simulink model "SP_Dynamic_17Okt_ExergyFlow"  (R2019b)
settings: Solver=FixedStepAuto  StartTime=0.0  StopTime=0  FixedStep=1/3600  RelTol=1e-3
model workspace (MAT data in the model file):
  AD = Simulink.Parameter
  AD.Value = [1; 1; 1; 23.3; 33.9; 32.8; 49.9; 50.5]
  AD.DataType = 'auto'
  AD.Dimensions = [8 1]
  AG = Simulink.Parameter
  AG.Value = [3.411e-06; 3.799e-07; 2.491e-07; 3.567e-07; 3.463e-07; 3.93e-07; 1.7e-07; 1.5e-07]
  AG.Description = 'Coefficient A to determine Enthalpy
    | MBtu/lb·°F'
  AG.DataType = 'auto'
  AG.Dimensions = [8 1]
  AH = Simulink.Parameter
  AH.Value = [1e-06; 1e-06; 1e-06; 9.6e-07; 5.73e-07; 6.52e-07; 5.15e-07; 4.71e-07]
  AH.Description = 'Coefficient C to determine Enthalpy
    | MBtu/lb·°F³'
  AH.DataType = 'auto'
  AH.Dimensions = [8 1]
  AV = Simulink.Parameter
  AV.Value = [1e-06; 1e-06; 1e-06; 8.67e-05; 0.00016; 0.00016; 0.000225; 0.000209]
  AV.DataType = 'auto'
  AV.Dimensions = [8 1]
  AVP = Simulink.Parameter
  AVP.Value = [0; 0; 0; 15.92; 16.35; 16.35; 16.43; 17.21]
  AVP.DataType = 'auto'
  AVP.Dimensions = [8 1]
  BCHL = Simulink.Parameter
  BCHL.Value = [0; 0; 0; 2118895; 2331760; 2492349; 2279927; 2994129]
  BCHL.DataType = 'auto'
  BCHL.Dimensions = [8 1]
  BCHV = Simulink.Parameter
  BCHV.Value = [254278; 948838; 625079; 1822034; 1979455; 2321416; 1491254; 1822996]
  BCHV.DataType = 'auto'
  BCHV.Dimensions = [8 1]
  BD = Simulink.Parameter
  BD.Value = [0; 0; 0; -0.07; -0.0957; -0.0995; -0.0191; -0.0541]
  BD.DataType = 'auto'
  BD.Dimensions = [8 1]
  BG = Simulink.Parameter
  BG.Value = [7.18e-10; 1.08e-09; 1.36e-11; 8.51e-10; 8.96e-10; 1.02e-09; 0; 0]
  BG.Description = 'Coefficient B to determine Enthalpy
    | MBtu/lb·°F²'
  BG.DataType = 'auto'
  BG.Dimensions = [8 1]
  BH = Simulink.Parameter
  BH.Value = [0; 0; 0; 8.7e-09; 2.41e-09; 2.18e-09; 5.65e-10; 8.7e-10]
  BH.Description = 'Coefficient B to determine Enthalpy
    | MBtu/lb·°F²'
  BH.DataType = 'auto'
  BH.Dimensions = [8 1]
  BVP = Simulink.Parameter
  BVP.Value = [0; 0; 0; -1444; -2114; -2114; -2748; -3318]
  BVP.DataType = 'auto'
  BVP.Dimensions = [8 1]
  CD = Simulink.Parameter
  CD.Value = [0; 0; 0; -0.0002; -0.000152; -0.000233; -0.000425; -0.00015]
  CD.DataType = 'auto'
  CD.Dimensions = [8 1]
  CG = Simulink.Parameter
  CG.Value = [6e-13; -3.98e-13; -3.93e-14; -3.12e-13; -3.27e-13; -3.12e-13; 0; 0]
  CG.DataType = 'auto'
  CG.Dimensions = [8 1]
  CH = Simulink.Parameter
  CH.Value = [0; 0; 0; 4.81e-11; 1.82e-11; 1.94e-11; 3.82e-12; 2.62e-12]
  CH.DataType = 'auto'
  CH.Dimensions = [8 1]
  CVP = Simulink.Parameter
  CVP.Value = [0; 0; 0; 259; 265.5; 265.5; 232.9; 249.6]
  CVP.DataType = 'auto'
  CVP.Dimensions = [8 1]
  XMW = Simulink.Parameter
  XMW.Value = [2; 25.4; 28; 32; 46; 48; 62; 76]
  XMW.Description = 'Molecular Weight of components lb/lb-mol'
  XMW.DataType = 'auto'
  XMW.Dimensions = [8 1]
undefined symbols (not defined in the file or in its folder): magnitude, SETPT, XMEAS, XMV
libraries: mylib x165, dspindex x17
(part 1 of 10)
settings Model: Creator=j3vos  LastModifiedBy=j3vos
settings DataIOCC: ReturnWorkspaceOutputs=off
settings DebuggingCC: ArithmeticOperatorsInVariantConditions=warning
settings SFSimCC: SimUseLocalCustomCode=off  CustomCodeUndefinedFunction=UseInterfaceOnly
settings RTWCC: RTWUseLocalCustomCode=off

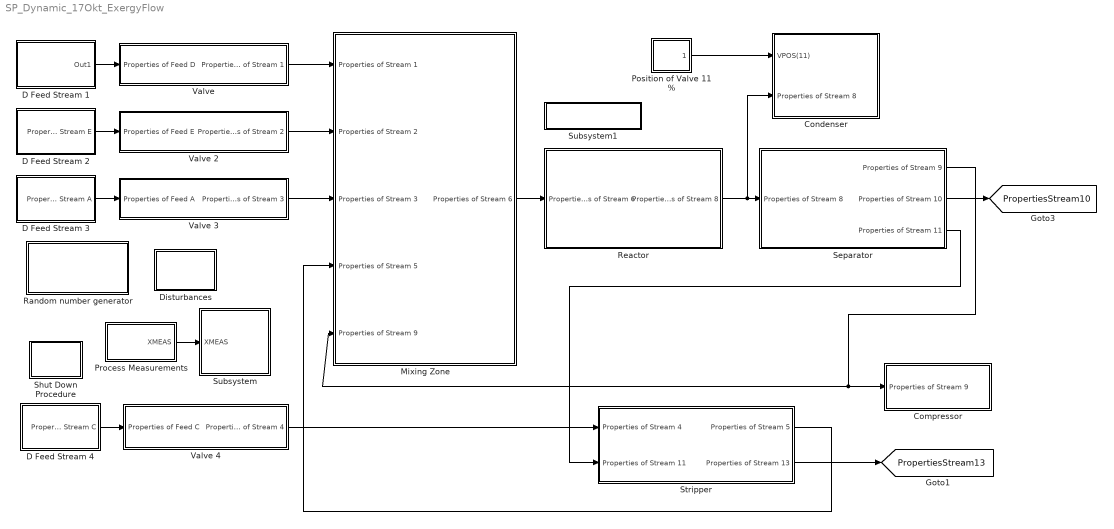
== system SP_Dynamic_17Okt_ExergyFlow ==
  Compressor : Subsystem
  Condenser : Subsystem
  D Feed Stream 1 : Subsystem  mask{XST1_A=0, XST1_B=0.0001, XST1_C=0, XST1_D=0.9999, XST1_E=0, XST1_F=0, XST1_G=0, XST1_H=0, TST1=45, VRNG1=400}
      mask prompts: XST1_A "Fraction of A in Stream 1"; XST1_B "Fraction of B in Stream 1"; XST1_C "Fraction of C in Stream 1"; XST1_D "Fraction of D in Stream 1"; XST1_E "Fraction of E in Stream 1"; XST1_F "Fraction of F in Stream 1"; XST1_G "Fraction of G in Stream 1"; XST1_H "Fraction of H in Stream 1"; TST1 "Temperature of Stream 1"; VRNG1 "Maximum flow of Stream 1"
      mask DialogControl DescTextVar Prompt: Enter the Composition, Temperature and Mass Flow of Feed Stream D entering the plant
      mask DialogControl ParameterGroupVar Prompt: Properties of Feed Stream D
      mask Display: color('Blue'),disp('Properties\nof\nFeed Stream D'),
  D Feed Stream 2 : Subsystem  mask{XST2_A=0, XST2_B=0, XST2_C=0, XST2_D=0, XST2_E=0.9999, XST2_F=0.0001, XST2_G=0, XST2_H=0, TST2=45, VRNG2=400}
      mask prompts: XST2_A "Fraction of A in Stream 2"; XST2_B "Fraction of B in Stream 2"; XST2_C "Fraction of C in Stream 2"; XST2_D "Fraction of D in Stream 2"; XST2_E "Fraction of E in Stream 2"; XST2_F "Fraction of F in Stream 2"; XST2_G "Fraction of G in Stream 2"; XST2_H "Fraction of H in Stream 2"; TST2 "Temperature of Stream 2"; VRNG2 "Maximum flow of Stream 2"
      mask DialogControl DescTextVar Prompt: Enter the Composition, Temperature and Mass Flow of Feed Stream E entering the plant
      mask DialogControl ParameterGroupVar Prompt: Properties of Feed Stream E
      mask Display: color('Red'),disp('Properties\nof\nFeed Stream E')
  D Feed Stream 3 : Subsystem  mask{XST3_A=0.9999, XST3_B=0.0001, XST3_C=0, XST3_D=0, XST3_E=0, XST3_F=0, XST3_G=0, XST3_H=0, TST3=45, VRNG3=100}
      mask prompts: XST3_A "Fraction of A in Stream 3"; XST3_B "Fraction of B in Stream 3"; XST3_C "Fraction of C in Stream 3"; XST3_D "Fraction of D in Stream 3"; XST3_E "Fraction of E in Stream 3"; XST3_F "Fraction of F in Stream 3"; XST3_G "Fraction of G in Stream 3"; XST3_H "Fraction of H in Stream 3"; TST3 "Temperature of Stream 3"; VRNG3 "Maximum flow of Stream 3"
      mask DialogControl DescTextVar Prompt: Enter the Composition, Temperature and Mass Flow of Feed Stream A entering the plant
      mask DialogControl ParameterGroupVar Prompt: Properties of Feed Stream A
      mask Display: color('Green'),disp('Properties\nof\nFeed Stream A')
  D Feed Stream 4 : Subsystem  mask{XST4_A=0.485, XST4_B=0.005, XST4_C=0.51, XST4_D=0, XST4_E=0, XST4_F=0, XST4_G=0, XST4_H=0, TST4=45, VRNG4=1500}
      mask prompts: XST4_A "Fraction of A in Stream 4"; XST4_B "Fraction of B in Stream 4"; XST4_C "Fraction of C in Stream 4"; XST4_D "Fraction of D in Stream 4"; XST4_E "Fraction of E in Stream 4"; XST4_F "Fraction of F in Stream 4"; XST4_G "Fraction of G in Stream 4"; XST4_H "Fraction of H in Stream 4"; TST4 "Temperature of Stream 4"; VRNG4 "Maximum flow of Stream 4"
      mask DialogControl DescTextVar Prompt: Enter the Composition, Temperature and Mass Flow of Feed Stream C entering the plant
      mask DialogControl ParameterGroupVar Prompt: Properties of Feed Stream C
      mask Display: color('Orange'),disp('Properties\nof\nFeed Stream C')
  Disturbances : Subsystem  mask{dd=1, IDV1=off, IDV2=off, IDV3=off, IDV4=off, IDV5=off, IDV6=off, IDV7=off, IDV8=off, IDV9=off, IDV10=off, IDV11=off, IDV12=off, IDV13=off, IDV14=off, IDV15=off, IDV16=off, IDV17=off, IDV18=off, IDV19=off, IDV20=off}
      mask prompts: dd "Simulation time when disturbances should be introduced"; IDV1 "IDV(1) - A/C feed ratio"; IDV2 "IDV(2) - B composition"; IDV3 "IDV(3) - D feed temperature"; IDV4 "IDV(4) - Reactor cooling water inlet temperature"; IDV5 "IDV(5) - Condenser cooling water inlet temperature"; IDV6 "IDV(6) - A feed loss"; IDV7 "IDV(7) - C header pressure loss (reduced availability)"; IDV8 "IDV(8) - A, B, C feed composition"; IDV9 "IDV(9) - D feed temperature"; IDV10 "IDV(10) - C feed temperature"; IDV11 "IDV(11) - Reactor cooling water inlet temperature"; IDV12 "IDV(12) - Condenser cooling water inlet temperature"; IDV13 "IDV(13) - Reaction kinetics"; IDV14 "IDV(14) - Reactor cooling water valve"; IDV15 "IDV(15) - Condenser cooling water valve"; IDV16 "IDV(16) - Unknown"; IDV17 "IDV(17) - Unknown"; IDV18 "IDV(18) - Unknown"; IDV19 "IDV(19) - Unknown"; IDV20 "IDV(20) - Unknown"
      mask DialogControl DescTextVar Prompt: Indicate if any disturbances are present (more than one can be ticked at a time)
      mask DialogControl ParameterGroupVar Prompt: Disturbances
      mask Display: color('Black'),disp('Disturbance\noff/on')
  Mixing Zone : Subsystem
  Position of Valve 11 % : Subsystem
  Process Measurements : Subsystem
  Random number generator : Subsystem  mask{gain_val=8322308324}
      mask prompts: gain_val "Random Number"
      mask init:
      | Gain=gain_val
      mask DialogControl DescTextVar Prompt: Enter a random number so that every runs results will differ
      mask DialogControl ParameterGroupVar Prompt: Random number generator
      mask Display: disp(['Random number:\n \n ',num2str(Gain)])
  Reactor : Subsystem
  Separator : Subsystem
  Shut Down Procedure : Subsystem
  Stripper : Subsystem
  Subsystem : Subsystem  mask{OPL=off, B=on, R=off, XMV1_0=63.05263039, XMV2_0=53.97970677, XMV3_0=24.64355755, XMV4_0=61.30192144, XMV5_0=22.21000000, XMV6_0=40.06374673, XMV7_0=38.10034370, XMV8_0=46.53415582, XMV9_0=47.44573456, XMV10_0=41.10581288, XMV11_0=18.11349055, XMV12_0=50.00000000}
      mask prompts: OPL "Open loop"; B "Braatz"; R "Ricker"; XMV1_0 "Initial value of XMV(1) - D Feed flow valve"; XMV2_0 "Initial value of XMV(2) - E Feed flow valve"; XMV3_0 "Initial value of XMV(3) - A Feed flow valve"; XMV4_0 "Initial value of XMV(4) - A and C Feed flow valve"; XMV5_0 "Initial value of XMV(5) - Compressor recycle valve"; XMV6_0 "Initial value of XMV(6) - Purge valve"; XMV7_0 "Initial value of XMV(7) - Separator liquid flow valve"; XMV8_0 "Initial value of XMV(8) - Stripper liquid product flow valve"; XMV9_0 "Initial value of XMV(9) - Stripper steam valve"; XMV10_0 "Initial value of XMV(10) - Reactor cooling water flow valve"; XMV11_0 "Initial value of XMV(11) - Condenser cooling water flow valve"; XMV12_0 "Initial value of XMV(12) - Agitator speed"
      mask DialogControl DescGroupVar Prompt: Manipulated variables
      mask DialogControl DescTextVar Prompt: Control loops for manipulated variables. Open loop is the original TEP process without any control. Only one loop can be selected for a run. The base case values are the initial values of the manipulated variables
      mask DialogControl ParameterGroupVar Prompt: Control strategy
      mask DialogControl Container6 Prompt: Base case values
      mask Display: color('Black'),disp('Control loop')
  Subsystem1 : Subsystem
      mask Display: color('Black'),disp('Exergy of streams')
  Valve : Subsystem
  Valve 2 : Subsystem
  Valve 3 : Subsystem
  Valve 4 : Subsystem
  tag scope: PropertiesStream10=global, PropertiesStream13=global
  wires:
  Position of Valve 11 %/1("YY(49) ") -> Condenser/1(VPOS(11))
  Valve/1(Properties of Stream 1) -> Mixing Zone/1(Properties of Stream 1)
  D Feed Stream 2/1("Properties of Feed Stream E ") -> Valve 2/1(Properties of Feed E)
  Valve 2/1(Properties of Stream 2) -> Mixing Zone/2(Properties of Stream 2)
  D Feed Stream 3/1("Properties of Feed Stream A ") -> Valve 3/1(Properties of Feed A)
  Valve 3/1(Properties of Stream 3) -> Mixing Zone/3(Properties of Stream 3)
  Stripper/1(Properties of Stream 5) -> Mixing Zone/4(Properties of Stream 5)
  Mixing Zone/1(Properties of Stream 6) -> Reactor/1(Properties of Stream 6)
  D Feed Stream 4/1("Properties of Feed Stream C ") -> Valve 4/1(Properties of Feed C)
  Valve 4/1(Properties of Stream 4) -> Stripper/1(Properties of Stream 4)
  Separator/3(Properties of Stream 11) -> Stripper/2(Properties of Stream 11)
  Reactor/1(Properties of Stream 8) -> Condenser/2(Properties of Stream 8), Separator/1(Properties of Stream 8)
  Separator/1(Properties of Stream 9) -> Mixing Zone/5(Properties of Stream 9), Compressor/1(Properties of Stream 9)
  D Feed Stream 1/1(Out1) -> Valve/1(Properties of Feed D)
  Process Measurements/1(XMEAS) -> Subsystem/1(XMEAS)
  Stripper/2(Properties of Stream 13) -> [PropertiesStream13]
  Separator/2(Properties of Stream 10) -> [PropertiesStream10]

== system SP_Dynamic_17Okt_ExergyFlow/Compressor ==
  Properties of Stream 9 : Inport
  "  " : Subsystem
  Bus Selector : BusSelector  OutputSignals=XMWS(9)
  CPDH Compressor work MBtu/h : Subsystem
  CPFLMX : Constant  Value=280275
  Subsystem : Subsystem
  Subsystem1 : Subsystem
  TKS Temperature of Separator K : Sum
  To Convert °C to K : Constant  Value=273.15
  tag scope: CPDH=global, FLMS=global
  wires:
  Subsystem1/1(FLCOEF) -> "  "/3(FLCOEF)
  Subsystem/1(PR) -> "  "/1(PR)
  CPFLMX/1 -> "  "/2(CPFLMX), Subsystem1/1(CPFLMX)
  CPDH Compressor work MBtu/h/1(CPDH) -> [CPDH]
  "  "/1(FLMS) -> [FLMS], CPDH Compressor work MBtu/h/1(FLMS)
  TKS Temperature of Separator K/1 -> CPDH Compressor work MBtu/h/2(TKS)
  [TCS] -> TKS Temperature of Separator K/1
  To Convert °C to K/1 -> TKS Temperature of Separator K/2
  Properties of Stream 9/1 -> Bus Selector/1
  Bus Selector/1 -> CPDH Compressor work MBtu/h/3("XMWS(9) ")  "<XMWS(9)>"

== system SP_Dynamic_17Okt_ExergyFlow/Condenser ==
  VPOS(11) : Inport
  Properties of Stream 8 : Inport  Port=2
  FWS Flow of cooling water to Condenser lb-mol/h : Subsystem
  Subsystem : Subsystem
  Subsystem1 : Subsystem
  "VRNG(11) Max flow of water through valve " : Constant  Value=1200
  tag scope: QUS=global
  wires:
  "VRNG(11) Max flow of water through valve "/1 -> FWS Flow of cooling water to Condenser lb-mol/h/2(VRNG(11))
  FWS Flow of cooling water to Condenser lb-mol/h/1(FWS) -> Subsystem1/1(FWS)
  VPOS(11)/1 -> FWS Flow of cooling water to Condenser lb-mol/h/1(VPOS(11))
  Subsystem/1("QUS ") -> Subsystem1/2(QUS), [QUS]
  Properties of Stream 8/1 -> Subsystem/1(Properties of Stream 8)
  Subsystem1/1("YY(38) ") -> Subsystem/2(In2)

== system SP_Dynamic_17Okt_ExergyFlow/D Feed Stream 1 ==
  Bus Creator : BusCreator  Inputs=4
  HST(1) Molar Enthalpy of Stream 1 MBtu/lb-mol : Subsystem
  TST(1) Temperature of Stream 1 °C : Subsystem
  VRNG(1) Max flow of Stream 1 through valve lb-mol/h : Constant  Value=VRNG1
  XST(I,1) Composition of Stream 1 : Constant  Value=[XST1_A;XST1_B;XST1_C;XST1_D;XST1_E;XST1_F;XST1_G;XST1_H]
  Out1 : Outport  VectorParamsAs1DForOutWhenUnconnected=off
  wires:
  XST(I,1) Composition of Stream 1/1 -> HST(1) Molar Enthalpy of Stream 1 MBtu/lb-mol/2(XST(I,1)), Bus Creator/1  "XST(I;1)"
  VRNG(1) Max flow of Stream 1 through valve lb-mol/h/1 -> Bus Creator/3  "VRNG(1)"
  HST(1) Molar Enthalpy of Stream 1 MBtu/lb-mol/1(HST(1)) -> Bus Creator/4  "HST(1)"
  TST(1) Temperature of Stream 1 °C/1(TST(1)) -> Bus Creator/2, HST(1) Molar Enthalpy of Stream 1 MBtu/lb-mol/1(TST(1))
  Bus Creator/1 -> Out1/1

== system SP_Dynamic_17Okt_ExergyFlow/D Feed Stream 2 ==
  Bus Creator : BusCreator  Inputs=4
  HST(2) Molar Enthalpy of Stream 2 MBtu/lb-mol : Subsystem
  TST(2) Temperature of Stream 2 °C : Constant  Value=TST2
  VRNG(2) Max flow of Stream 2 through valve lb-mol/h : Constant  Value=VRNG2
  XST(I,2) Composition of Stream 2 : Constant  Value=[XST2_A;XST2_B;XST2_C;XST2_D;XST2_E;XST2_F;XST2_G;XST2_H]
  "Properties of Feed Stream E " : Outport  VectorParamsAs1DForOutWhenUnconnected=off
  wires:
  XST(I,2) Composition of Stream 2/1 -> HST(2) Molar Enthalpy of Stream 2 MBtu/lb-mol/2(XST(I,2)), Bus Creator/1  "XST(I;2)"
  TST(2) Temperature of Stream 2 °C/1 -> HST(2) Molar Enthalpy of Stream 2 MBtu/lb-mol/1(TST(2)), Bus Creator/2  "TST(2)"
  VRNG(2) Max flow of Stream 2 through valve lb-mol/h/1 -> Bus Creator/3  "VRNG(2)"
  Bus Creator/1 -> "Properties of Feed Stream E "/1
  HST(2) Molar Enthalpy of Stream 2 MBtu/lb-mol/1(HST(2)) -> Bus Creator/4  "HST(2)"

== system SP_Dynamic_17Okt_ExergyFlow/D Feed Stream 3 ==
  Bus Creator : BusCreator  Inputs=4
  HST(3) Molar Enthalpy of Stream 3 MBtu/lb-mol : Subsystem
  TST(3) Temperature of Stream 3 °C : Constant  Value=TST3
  VRNG(3) Max flow of Stream 3 through valve lb-mol/h : Constant  Value=VRNG3
  XST(I,3) Composition of Stream 3 : Constant  Value=[XST3_A;XST3_B;XST3_C;XST3_D;XST3_E;XST3_F;XST3_G;XST3_H]
  "Properties of Feed Stream A " : Outport  VectorParamsAs1DForOutWhenUnconnected=off
  wires:
  XST(I,3) Composition of Stream 3/1 -> HST(3) Molar Enthalpy of Stream 3 MBtu/lb-mol/2(XST(I,3)), Bus Creator/1  "XST(I;3)"
  TST(3) Temperature of Stream 3 °C/1 -> HST(3) Molar Enthalpy of Stream 3 MBtu/lb-mol/1(TST(3)), Bus Creator/2  "TST(3)"
  VRNG(3) Max flow of Stream 3 through valve lb-mol/h/1 -> Bus Creator/3  "VRNG(3)"
  HST(3) Molar Enthalpy of Stream 3 MBtu/lb-mol/1(HST(3)) -> Bus Creator/4  "HST(3)"
  Bus Creator/1 -> "Properties of Feed Stream A "/1

== system SP_Dynamic_17Okt_ExergyFlow/D Feed Stream 4 ==
  note: TST(4)
      | Temperature of Stream 4
      | °C
  Bus Creator : BusCreator  Inputs=4
  Bus Selector : BusSelector  OutputSignals=TESUB8(1),TESUB8(2)
  Bus Selector1 : BusSelector  OutputSignals=IDV(1),IDV(2)
  Bus Selector2 : BusSelector  OutputSignals=TESUB8(4)
  Gain : Gain
  HST(4) Molar Enthalpy of Stream 4 MBtu/lb-mol : Subsystem
  VRNG(4) Max flow of Stream 4 through valve lb-mol/h : Constant  Value=VRNG4
  "XST(I;4) Composition of Stream 4 " : Subsystem
  "Properties of Feed Stream C " : Outport  VectorParamsAs1DForOutWhenUnconnected=off
  wires:
  "XST(I;4) Composition of Stream 4 "/1(XST(I;4)) -> HST(4) Molar Enthalpy of Stream 4 MBtu/lb-mol/2(XST(I,4)), Bus Creator/1  "XST(I;4)"
  Bus Selector2/1 -> HST(4) Molar Enthalpy of Stream 4 MBtu/lb-mol/1(TST(4)), Gain/1  "<TESUB8(4)>"
  VRNG(4) Max flow of Stream 4 through valve lb-mol/h/1 -> Bus Creator/3  "VRNG(4)"
  Bus Creator/1 -> "Properties of Feed Stream C "/1
  HST(4) Molar Enthalpy of Stream 4 MBtu/lb-mol/1(HST(4)) -> Bus Creator/4  "HST(4)"
  Bus Selector/2 -> "XST(I;4) Composition of Stream 4 "/2(TESUB8(2))  "<TESUB8(2)>"
  [TESUB8] -> Bus Selector2/1, Bus Selector/1
  Bus Selector/1 -> "XST(I;4) Composition of Stream 4 "/1(TESUB8(1))  "<TESUB8(1)>"
  [IDV] -> Bus Selector1/1
  Bus Selector1/1 -> "XST(I;4) Composition of Stream 4 "/3(IDV(1))  "<IDV(1)>"
  Bus Selector1/2 -> "XST(I;4) Composition of Stream 4 "/4(IDV(2))  "<IDV(2)>"
  Gain/1 -> Bus Creator/2  "TST(4)"

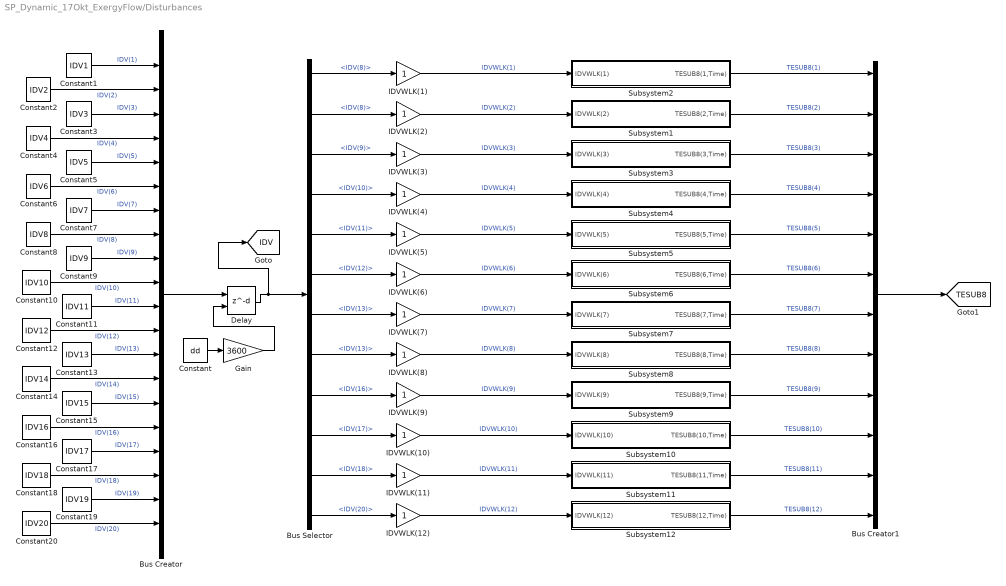
== system SP_Dynamic_17Okt_ExergyFlow/Disturbances ==
  Bus Creator : BusCreator  Inputs=20
  Bus Creator1 : BusCreator  Inputs=12
  Bus Selector : BusSelector  OutputSignals=IDV(8),IDV(8),IDV(9),IDV(10),IDV(11),IDV(12),IDV(13),IDV(13),IDV(16),IDV(17),IDV(18),IDV(20)
  Constant : Constant  Value=dd
  Constant1 : Constant  Value=IDV1
  Constant10 : Constant  Value=IDV10
  Constant11 : Constant  Value=IDV11
  Constant12 : Constant  Value=IDV12
  Constant13 : Constant  Value=IDV13
  Constant14 : Constant  Value=IDV14
  Constant15 : Constant  Value=IDV15
  Constant16 : Constant  Value=IDV16
  Constant17 : Constant  Value=IDV17
  Constant18 : Constant  Value=IDV18
  Constant19 : Constant  Value=IDV19
  Constant2 : Constant  Value=IDV2
  Constant20 : Constant  Value=IDV20
  Constant3 : Constant  Value=IDV3
  Constant4 : Constant  Value=IDV4
  Constant5 : Constant  Value=IDV5
  Constant6 : Constant  Value=IDV6
  Constant7 : Constant  Value=IDV7
  Constant8 : Constant  Value=IDV8
  Constant9 : Constant  Value=IDV9
  Delay : Delay  DelayLengthSource=Input port  DelayLength=1  DelayLengthUpperLimit=dd*3600  InitialCondition=0
      settings: InputPortMap=u0,p1
  Gain : Gain  Gain=3600
  IDVWLK(1) : Gain
  IDVWLK(10) : Gain
  IDVWLK(11) : Gain
  IDVWLK(12) : Gain
  IDVWLK(2) : Gain
  IDVWLK(3) : Gain
  IDVWLK(4) : Gain
  IDVWLK(5) : Gain
  IDVWLK(6) : Gain
  IDVWLK(7) : Gain
  IDVWLK(8) : Gain
  IDVWLK(9) : Gain
  Subsystem1 : Subsystem
  Subsystem10 : Subsystem
  Subsystem11 : Subsystem
  Subsystem12 : Subsystem
  Subsystem2 : Subsystem
  Subsystem3 : Subsystem
  Subsystem4 : Subsystem
  Subsystem5 : Subsystem
  Subsystem6 : Subsystem
  Subsystem7 : Subsystem
  Subsystem8 : Subsystem
  Subsystem9 : Subsystem
  tag scope: IDV=global, TESUB8=global
  wires:
  Constant1/1 -> Bus Creator/1  "IDV(1)"
  Constant2/1 -> Bus Creator/2  "IDV(2)"
  Constant3/1 -> Bus Creator/3  "IDV(3)"
  Constant4/1 -> Bus Creator/4  "IDV(4)"
  Constant5/1 -> Bus Creator/5  "IDV(5)"
  Constant6/1 -> Bus Creator/6  "IDV(6)"
  Constant7/1 -> Bus Creator/7  "IDV(7)"
  Constant8/1 -> Bus Creator/8  "IDV(8)"
  Constant9/1 -> Bus Creator/9  "IDV(9)"
  Constant10/1 -> Bus Creator/10  "IDV(10)"
  Constant11/1 -> Bus Creator/11  "IDV(11)"
  Constant12/1 -> Bus Creator/12  "IDV(12)"
  Constant13/1 -> Bus Creator/13  "IDV(13)"
  Constant14/1 -> Bus Creator/14  "IDV(14)"
  Constant15/1 -> Bus Creator/15  "IDV(15)"
  Constant16/1 -> Bus Creator/16  "IDV(16)"
  Constant17/1 -> Bus Creator/17  "IDV(17)"
  Constant18/1 -> Bus Creator/18  "IDV(18)"
  Constant19/1 -> Bus Creator/19  "IDV(19)"
  Constant20/1 -> Bus Creator/20  "IDV(20)"
  Bus Selector/5 -> IDVWLK(5)/1  "<IDV(11)>"
  Bus Selector/7 -> IDVWLK(7)/1  "<IDV(13)>"
  Bus Selector/9 -> IDVWLK(9)/1  "<IDV(16)>"
  Subsystem6/1(TESUB8(6,Time)) -> Bus Creator1/6  "TESUB8(6)"
  Subsystem3/1(TESUB8(3,Time)) -> Bus Creator1/3  "TESUB8(3)"
  Subsystem2/1(TESUB8(1,Time)) -> Bus Creator1/1  "TESUB8(1)"
  IDVWLK(10)/1 -> Subsystem10/1(IDVWLK(10))  "IDVWLK(10)"
  Subsystem7/1(TESUB8(7,Time)) -> Bus Creator1/7  "TESUB8(7)"
  Bus Selector/2 -> IDVWLK(2)/1  "<IDV(8)>"
  Subsystem8/1(TESUB8(8,Time)) -> Bus Creator1/8  "TESUB8(8)"
  Subsystem4/1(TESUB8(4,Time)) -> Bus Creator1/4  "TESUB8(4)"
  Bus Creator1/1 -> [TESUB8]
  Subsystem1/1(TESUB8(2,Time)) -> Bus Creator1/2  "TESUB8(2)"
  Bus Selector/12 -> IDVWLK(12)/1  "<IDV(20)>"
  IDVWLK(6)/1 -> Subsystem6/1(IDVWLK(6))  "IDVWLK(6)"
  IDVWLK(3)/1 -> Subsystem3/1(IDVWLK(3))  "IDVWLK(3)"
  IDVWLK(1)/1 -> Subsystem2/1(IDVWLK(1))  "IDVWLK(1)"
  Subsystem5/1(TESUB8(5,Time)) -> Bus Creator1/5  "TESUB8(5)"
  IDVWLK(9)/1 -> Subsystem9/1(IDVWLK(9))  "IDVWLK(9)"
  Bus Selector/1 -> IDVWLK(1)/1  "<IDV(8)>"
  Bus Selector/6 -> IDVWLK(6)/1  "<IDV(12)>"
  Bus Selector/4 -> IDVWLK(4)/1  "<IDV(10)>"
  IDVWLK(5)/1 -> Subsystem5/1(IDVWLK(5))  "IDVWLK(5)"
  Bus Selector/8 -> IDVWLK(8)/1  "<IDV(13)>"
  IDVWLK(2)/1 -> Subsystem1/1(IDVWLK(2))  "IDVWLK(2)"
  IDVWLK(8)/1 -> Subsystem8/1(IDVWLK(8))  "IDVWLK(8)"
  Bus Selector/3 -> IDVWLK(3)/1  "<IDV(9)>"
  Bus Selector/10 -> IDVWLK(10)/1  "<IDV(17)>"
  IDVWLK(7)/1 -> Subsystem7/1(IDVWLK(7))  "IDVWLK(7)"
  Bus Selector/11 -> IDVWLK(11)/1  "<IDV(18)>"
  Subsystem9/1(TESUB8(9,Time)) -> Bus Creator1/9  "TESUB8(9)"
  IDVWLK(4)/1 -> Subsystem4/1(IDVWLK(4))  "IDVWLK(4)"
  Bus Creator/1 -> Delay/1
  Subsystem10/1(TESUB8(10,Time)) -> Bus Creator1/10  "TESUB8(10)"
  Subsystem11/1(TESUB8(11,Time)) -> Bus Creator1/11  "TESUB8(11)"
  IDVWLK(11)/1 -> Subsystem11/1(IDVWLK(11))  "IDVWLK(11)"
  Subsystem12/1(TESUB8(12,Time)) -> Bus Creator1/12  "TESUB8(12)"
  IDVWLK(12)/1 -> Subsystem12/1(IDVWLK(12))  "IDVWLK(12)"
  Delay/1 -> Bus Selector/1, [IDV]
  Constant/1 -> Gain/1
  Gain/1 -> Delay/2

== system SP_Dynamic_17Okt_ExergyFlow/Mixing Zone ==
  Properties of Stream 1 : Inport
  Properties of Stream 2 : Inport  Port=2
  Properties of Stream 3 : Inport  Port=3
  Properties of Stream 5 : Inport  Port=4
  Properties of Stream 9 : Inport  Port=5
  Bus Creator : BusCreator  Inputs=2
  ETV Internal energy of Mixing zone Btu : Gain
  Holdup of Components in Mixing Zone : Subsystem
  Internal energy of mixing zone : Subsystem
  PTV Total pressure of Mixing zone mmHg : Subsystem
  Stream 6 : Subsystem
  "TCV Initial Temperature in Mixing zone °C " : Subsystem
  Properties of Stream 6 : Outport  VectorParamsAs1DForOutWhenUnconnected=off
  tag scope: PTV=global, PropertiesStream6=global
  wires:
  "TCV Initial Temperature in Mixing zone °C "/1(TCV) -> PTV Total pressure of Mixing zone mmHg/2(TCV), Stream 6/2(TST(6))
  Internal energy of mixing zone/1("YY(36) ") -> ETV Internal energy of Mixing zone Btu/1
  ETV Internal energy of Mixing zone Btu/1 -> "TCV Initial Temperature in Mixing zone °C "/2(ETV)
  Properties of Stream 1/1 -> Holdup of Components in Mixing Zone/1(Properties of Stream 1), Internal energy of mixing zone/1(Properties of Stream 1)
  Properties of Stream 2/1 -> Internal energy of mixing zone/2(Properties of Stream 2), Holdup of Components in Mixing Zone/2(Properties of Stream 2)
  Properties of Stream 3/1 -> Internal energy of mixing zone/3(Properties of Stream 3), Holdup of Components in Mixing Zone/3(Properties of Stream 3)
  Stream 6/1(Properties of Stream 6) -> Bus Creator/1, Properties of Stream 6/1
  Properties of Stream 5/1 -> Internal energy of mixing zone/4(Properties of Stream 5), Holdup of Components in Mixing Zone/4(Properties of Stream 5)
  Properties of Stream 9/1 -> Internal energy of mixing zone/5(Properties of Stream 9), Holdup of Components in Mixing Zone/5(Properties of Stream 9)
  Holdup of Components in Mixing Zone/1(XVV) -> Stream 6/1(XST(I,6)), "TCV Initial Temperature in Mixing zone °C "/3(XVV)
  Holdup of Components in Mixing Zone/2(UTVV) -> PTV Total pressure of Mixing zone mmHg/1(UTVV), "TCV Initial Temperature in Mixing zone °C "/1(UTVV)
  PTV Total pressure of Mixing zone mmHg/1(PTV) -> Bus Creator/2, [PTV]  "PTV"
  Bus Creator/1 -> [PropertiesStream6]

== system SP_Dynamic_17Okt_ExergyFlow/Position of Valve 11 % ==
  Bus Selector : BusSelector  OutputSignals=XMV(11)
  Bus Selector1 : BusSelector  OutputSignals=IDV(15)
  Control valve : mylib/Control valve  SystemSampleTime=-1  Latency=0  AutoFrameSizeCalculation=off
  Divide : Product  Inputs=*/
  Subtract : Sum  Inputs=+-
  VTAU(11) : Constant  Value=5/3600
  YP(49) : Integrator  InitialConditionSource=external
  YY(49) : Constant  Value=18.11349055
  "YY(49) " : Outport  PortDimensions=1  VectorParamsAs1DForOutWhenUnconnected=off
  wires:
  YP(49)/1 -> Subtract/2, "YY(49) "/1  "VPOS(11)"
  Subtract/1 -> Divide/1
  Control valve/1 -> Subtract/1
  VTAU(11)/1 -> Divide/2
  Divide/1 -> YP(49)/1
  YY(49)/1 -> YP(49)/2
  [XMV] -> Bus Selector/1
  Bus Selector/1 -> Control valve/1  "<XMV(11)>"
  Bus Selector1/1 -> Control valve/2  "<IDV(15)>"
  [IDV] -> Bus Selector1/1

== system SP_Dynamic_17Okt_ExergyFlow/Process Measurements ==
  Bus Creator1 : BusCreator  Inputs=10
  Compressor Work : Subsystem
  Condenser Cooling Outlet Water Temperature : Subsystem
  Feed Streams : Subsystem
  Product analysis : Subsystem
  Purge gas analysis : Subsystem
  Reactor Cooling Outlet Water Temperature : Subsystem
  Reactor feed analysis : Subsystem
  Subsystem3 : Subsystem
  Subsystem4 : Subsystem
  Subsystem5 : Subsystem
  To Workspace : ToWorkspace  VariableName=XMEAS20  SampleTime=-1
  XMEAS : Outport  VectorParamsAs1DForOutWhenUnconnected=off
  wires:
  Bus Creator1/1 -> XMEAS/1, To Workspace/1
  Feed Streams/1(XMEASF) -> Bus Creator1/1
  Subsystem3/1(Reactor) -> Bus Creator1/2
  Subsystem4/1(Separator) -> Bus Creator1/3
  Subsystem5/1(Stripper) -> Bus Creator1/4
  Product analysis/1(XMEAS) -> Bus Creator1/10
  Purge gas analysis/1(XMEASP) -> Bus Creator1/9
  Reactor feed analysis/1(XMEASR) -> Bus Creator1/8
  Compressor Work/1("XMEAS(20) ") -> Bus Creator1/5
  Reactor Cooling Outlet Water Temperature/1(XMEAS(21)) -> Bus Creator1/6
  Condenser Cooling Outlet Water Temperature/1(XMEAS(22)) -> Bus Creator1/7

== system SP_Dynamic_17Okt_ExergyFlow/Random number generator ==
  Constant : Constant
  Delay : Delay  DelayLength=1  InitialConditionSource=Input port  InitialCondition=0
      settings: InputPortMap=u0,p4
  Display{1..6} (6 alike) : Display
  Disturbances I=1-9 : Subsystem
  Disturbances I=10-12 : Subsystem
  Gain : Gain  Gain=Gain
  Process Measurements XMEAS(I) I=1-22 : Subsystem
  Process Measurements XMEAS(I) I=23-36 : Subsystem
  Process Measurements XMEAS(I) I=37-41 : Subsystem
  wires:
  Constant/1 -> Gain/1
  Disturbances I=10-12/1(G3) -> Display2/1, Process Measurements XMEAS(I) I=1-22/1(G2)
  Process Measurements XMEAS(I) I=37-41/1(G5) -> Delay/1, Display4/1
  Gain/1 -> Delay/2
  Process Measurements XMEAS(I) I=1-22/1(G3) -> Process Measurements XMEAS(I) I=23-36/1(G3), Display5/1
  Process Measurements XMEAS(I) I=23-36/1(G4) -> Display3/1, Process Measurements XMEAS(I) I=37-41/1(G4)
  Disturbances I=1-9/1(G1) -> Display1/1, Disturbances I=10-12/1(G2)
  Delay/1 -> Display6/1, Disturbances I=1-9/1(G)

== system SP_Dynamic_17Okt_ExergyFlow/Reactor ==
  Properties of Stream 6 : Inport
  Bus Creator : BusCreator  Inputs=2
  Holdup of Components in Reactor : Subsystem
  Internal energy of reactor : Subsystem
  Pressure of Reactor : Subsystem
  Reaction Rates : Subsystem
  Reactor Heat exchanger : Subsystem
  Stream 8 : Subsystem
  "TCR Initial Temperature in Reactor °C " : Subsystem
  Total Vapour Component Holdup in Reactor : Subsystem
  Vapour Component Fraction in Reactor : Subsystem
  Volume of Reactor : Subsystem
  Properties of Stream 8 : Outport  VectorParamsAs1DForOutWhenUnconnected=off
  tag scope: PTR=global, PropertiesStream8=global, TCR=global, VLR=global
  wires:
  Holdup of Components in Reactor/1(UTLR) -> Volume of Reactor/2(UTLR), "TCR Initial Temperature in Reactor °C "/1(UTLR)
  Internal energy of reactor/1("YY(9) ") -> "TCR Initial Temperature in Reactor °C "/2(ETR)  "ETR Internal energy of reactor MBtu"
  Stream 8/1(Properties of Stream 8) -> Bus Creator/1, Properties of Stream 8/1
  Reactor Heat exchanger/1(QUR) -> Internal energy of reactor/2(QUR)
  Properties of Stream 6/1 -> Holdup of Components in Reactor/2(Properties of Stream 6), Internal energy of reactor/3(Properties of Stream 6)
  Reaction Rates/1("RH ") -> Internal energy of reactor/1(RH)
  Reaction Rates/2(CRXR) -> Holdup of Components in Reactor/1(CRXR)
  Holdup of Components in Reactor/2(XLR) -> Pressure of Reactor/1(XLR), "TCR Initial Temperature in Reactor °C "/3(XLR), Volume of Reactor/1(XLR)
  Holdup of Components in Reactor/3(UCVR) -> Pressure of Reactor/3(UCVR)
  Pressure of Reactor/2(PPR) -> Reaction Rates/2(PPR), Vapour Component Fraction in Reactor/1(PPR)
  Pressure of Reactor/1(PTR) -> Bus Creator/2, [PTR]  "PTR"
  "TCR Initial Temperature in Reactor °C "/1(TCR) -> Stream 8/1(TST(8)), [TCR]
  Volume of Reactor/1(VVR) -> Reaction Rates/1(VVR), Total Vapour Component Holdup in Reactor/1(VVR), Pressure of Reactor/2(VVR)
  Vapour Component Fraction in Reactor/1(XVR) -> Stream 8/2(XTS(I,8)), Total Vapour Component Holdup in Reactor/2(XVR)
  Volume of Reactor/2(VLR) -> [VLR]
  Bus Creator/1 -> [PropertiesStream8]

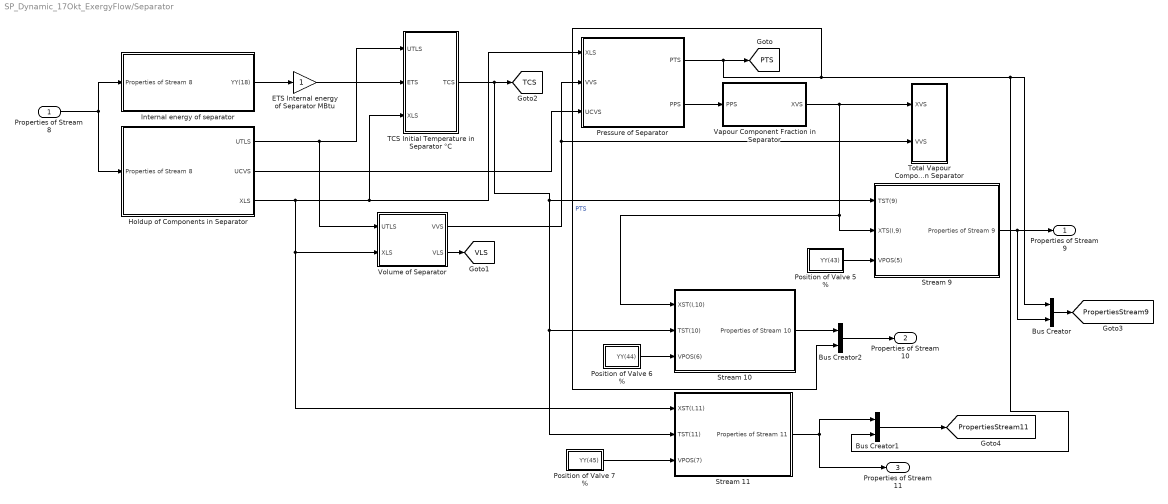
== system SP_Dynamic_17Okt_ExergyFlow/Separator ==
  Properties of Stream 8 : Inport
  Bus Creator : BusCreator  Inputs=2
  Bus Creator1 : BusCreator  Inputs=2
  Bus Creator2 : BusCreator  Inputs=2
  ETS Internal energy of Separator MBtu : Gain
  Holdup of Components in Separator : Subsystem
  Internal energy of separator : Subsystem
  Position of Valve 5 % : Subsystem
  Position of Valve 6 % : Subsystem
  Position of Valve 7 % : Subsystem
  Pressure of Separator : Subsystem
  Stream 10 : Subsystem
  Stream 11 : Subsystem
  Stream 9 : Subsystem
  "TCS Initial Temperature in Separator °C " : Subsystem
  Total Vapour Component Holdup in Separator : Subsystem
  Vapour Component Fraction in Separator : Subsystem
  Volume of Separator : Subsystem
  Properties of Stream 9 : Outport  VectorParamsAs1DForOutWhenUnconnected=off
  Properties of Stream 10 : Outport  Port=2  VectorParamsAs1DForOutWhenUnconnected=off
  Properties of Stream 11 : Outport  Port=3  VectorParamsAs1DForOutWhenUnconnected=off
  tag scope: PTS=global, PropertiesStream11=global, PropertiesStream9=global, TCS=global, VLS=global
  wires:
  Internal energy of separator/1("YY(18) ") -> ETS Internal energy of Separator MBtu/1
  Stream 9/1(Properties of Stream 9) -> Bus Creator/2, Properties of Stream 9/1
  Stream 11/1(Properties of Stream 11) -> Bus Creator1/1, Properties of Stream 11/1
  Holdup of Components in Separator/1(UTLS) -> Volume of Separator/1(UTLS), "TCS Initial Temperature in Separator °C "/1(UTLS)
  Holdup of Components in Separator/3(XLS) -> "TCS Initial Temperature in Separator °C "/3(XLS), Pressure of Separator/1(XLS), Stream 11/1(XST(I,11)), Volume of Separator/2(XLS)
  Volume of Separator/1(VVS) -> Pressure of Separator/2(VVS), Total Vapour Component Holdup in Separator/2(VVS)
  Volume of Separator/2(VLS) -> [VLS]
  Pressure of Separator/1(PTS) -> Bus Creator2/2, Bus Creator1/2, Bus Creator/1, [PTS]  "PTS"
  Holdup of Components in Separator/2(UCVS) -> Pressure of Separator/3(UCVS)
  Vapour Component Fraction in Separator/1(XVS) -> Stream 10/1(XST(I,10)), Stream 9/2(XTS(I,9)), Total Vapour Component Holdup in Separator/1(XVS)
  Pressure of Separator/2(PPS) -> Vapour Component Fraction in Separator/1(PPS)
  Properties of Stream 8/1 -> Internal energy of separator/1(Properties of Stream 8), Holdup of Components in Separator/1(Properties of Stream 8)
  Position of Valve 5 %/1("YY(43) ") -> Stream 9/3(VPOS(5))
  Position of Valve 6 %/1("YY(44) ") -> Stream 10/3(VPOS(6))
  Position of Valve 7 %/1("YY(45) ") -> Stream 11/3(VPOS(7))
  ETS Internal energy of Separator MBtu/1 -> "TCS Initial Temperature in Separator °C "/2(ETS)
  "TCS Initial Temperature in Separator °C "/1(TCS) -> [TCS], Stream 11/2(TST(11)), Stream 10/2(TST(10)), Stream 9/1(TST(9))
  Bus Creator/1 -> [PropertiesStream9]
  Bus Creator1/1 -> [PropertiesStream11]
  Stream 10/1(Properties of Stream 10) -> Bus Creator2/1
  Bus Creator2/1 -> Properties of Stream 10/1

== system SP_Dynamic_17Okt_ExergyFlow/Shut Down Procedure ==
  Product : Product  Inputs=8  OutDataTypeStr=double
  Reactor Level to High : Subsystem
  Reactor Level to Low : Subsystem
  Reactor Presssure to High : Subsystem
  Reactor Temperature to High : Subsystem
  Separator Level to High : Subsystem
  Separator Level to Low : Subsystem
  Stripper Level to High : Subsystem
  Stripper Level to Low : Subsystem
  tag scope: ISD=global
  wires:
  [VLR] -> Reactor Level to Low/1(VLR), Reactor Level to High/1(VLR)
  [VLS] -> Separator Level to Low/1(VLS), Separator Level to High/1(VLS)
  [VLC] -> Stripper Level to Low/1(VLC), Stripper Level to High/1(VLC)
  Product/1 -> [ISD]
  Reactor Presssure to High/1(ISD) -> Product/1
  Reactor Temperature to High/1(ISD) -> Product/2
  Reactor Level to High/1(ISD) -> Product/3
  Reactor Level to Low/1(ISD) -> Product/4
  Separator Level to High/1(ISD) -> Product/5
  Separator Level to Low/1(ISD) -> Product/6
  Stripper Level to High/1(ISD) -> Product/7
  Stripper Level to Low/1(ISD) -> Product/8

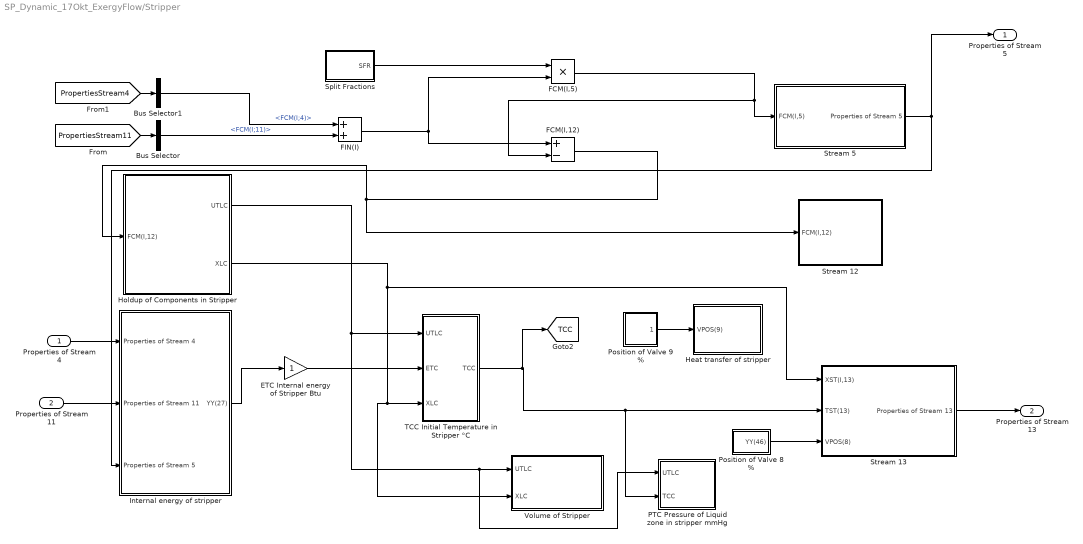
== system SP_Dynamic_17Okt_ExergyFlow/Stripper ==
  Properties of Stream 4 : Inport
  Properties of Stream 11 : Inport  Port=2
  Bus Selector : BusSelector  OutputSignals=signal1.FCM(I;11)
  Bus Selector1 : BusSelector  OutputSignals=FCM(I;4)
  ETC Internal energy of Stripper Btu : Gain
  FCM(I,12) : Sum  Inputs=+-
  FCM(I,5) : Product
  FIN(I) : Sum
  Heat transfer of stripper : Subsystem
  Holdup of Components in Stripper : Subsystem
  Internal energy of stripper : Subsystem
  PTC Pressure of Liquid zone in stripper mmHg : Subsystem
  Position of Valve 8 % : Subsystem
  Position of Valve 9 % : Subsystem
  Split Fractions : Subsystem
  Stream 12 : Subsystem
  Stream 13 : Subsystem
  Stream 5 : Subsystem
  "TCC Initial Temperature in Stripper °C " : Subsystem
  Volume of Stripper : Subsystem
  Properties of Stream 5 : Outport  VectorParamsAs1DForOutWhenUnconnected=off
  Properties of Stream 13 : Outport  Port=2  VectorParamsAs1DForOutWhenUnconnected=off
  tag scope: TCC=global
  wires:
  Holdup of Components in Stripper/1(UTLC) -> PTC Pressure of Liquid zone in stripper mmHg/1(UTLC), Volume of Stripper/1(UTLC), "TCC Initial Temperature in Stripper °C "/1(UTLC)
  Internal energy of stripper/1("YY(27) ") -> ETC Internal energy of Stripper Btu/1
  ETC Internal energy of Stripper Btu/1 -> "TCC Initial Temperature in Stripper °C "/2(ETC)
  "TCC Initial Temperature in Stripper °C "/1(TCC) -> [TCC], PTC Pressure of Liquid zone in stripper mmHg/2(TCC), Stream 13/2(TST(13))
  FIN(I)/1 -> FCM(I,12)/1, FCM(I,5)/2
  FCM(I,5)/1 -> FCM(I,12)/2, Stream 5/1(FCM(I,5))
  FCM(I,12)/1 -> Holdup of Components in Stripper/1("FCM(I,12) "), Stream 12/1(FCM(I,12))
  Stream 13/1(Properties of Stream 13) -> Properties of Stream 13/1
  Stream 5/1(Properties of Stream 5) -> Properties of Stream 5/1, Internal energy of stripper/3(Properties of Stream 5)
  Properties of Stream 4/1 -> Internal energy of stripper/1(Properties of Stream 4)
  Properties of Stream 11/1 -> Internal energy of stripper/2(Properties of Stream 11)
  Holdup of Components in Stripper/2(XLC) -> "TCC Initial Temperature in Stripper °C "/3(XLC), Volume of Stripper/2(XLC), Stream 13/1(XST(I,13))
  Position of Valve 9 %/1("YY(47) ") -> Heat transfer of stripper/1(VPOS(9))
  Split Fractions/1(SFR) -> FCM(I,5)/1
  [PropertiesStream11] -> Bus Selector/1
  Bus Selector/1 -> FIN(I)/2  "<FCM(I;11)>"
  [PropertiesStream4] -> Bus Selector1/1
  Bus Selector1/1 -> FIN(I)/1  "<FCM(I;4)>"
  Position of Valve 8 %/1("YY(46) ") -> Stream 13/3(VPOS(8))

== system SP_Dynamic_17Okt_ExergyFlow/Subsystem ==
  XMEAS : Inport
  Braatz : Subsystem
  Constant : Constant  Value=OPL
  Constant1 : Constant  Value=B
  Constant2 : Constant  Value=R
  If : If  NumInputs=3  IfExpression=u1 == 1  ElseIfExpressions=u2 == 1, u3 == 1  ShowElse=off
  If Action Subsystem : Subsystem  TreatAsAtomicUnit=on
  If Action Subsystem1 : Subsystem  TreatAsAtomicUnit=on
  If Action Subsystem2 : Subsystem  TreatAsAtomicUnit=on
  Merge : Merge  Inputs=3
  Open loop : Subsystem
  Ricker : Subsystem
  Scope : Scope
  Subsystem : Subsystem
      mask Display: color('Black'),disp('Multi loop\nselection')
  To Workspace : ToWorkspace  VariableName=XMV20  SampleTime=-1
  tag scope: XMV=global
  wires:
  Constant/1 -> Subsystem/1(OPL), If/1
  Constant1/1 -> Subsystem/2(B), If/2
  Constant2/1 -> Subsystem/3(R), If/3
  Merge/1 -> Scope/1, To Workspace/1, [XMV]
  If/1 -> If Action Subsystem/Action
  Open loop/1(XMV) -> If Action Subsystem/1(In1)
  If Action Subsystem1/1(Out1) -> Merge/2
  If/2 -> If Action Subsystem1/Action
  If/3 -> If Action Subsystem2/Action
  If Action Subsystem/1(Out1) -> Merge/1
  If Action Subsystem2/1(Out1) -> Merge/3
  Braatz/1(XMV) -> If Action Subsystem1/1(In1)
  Ricker/1(XMV) -> If Action Subsystem2/1(In1)
  XMEAS/1 -> Braatz/1(XMEAS)

== system SP_Dynamic_17Okt_ExergyFlow/Subsystem1 ==
  Bus Creator7 : BusCreator  Inputs=7
  Subsystem : Subsystem
  Subsystem1 : Subsystem
  Subsystem2 : Subsystem
  Subsystem3 : Subsystem
  Subsystem4 : Subsystem
  Subsystem5 : Subsystem
  Subsystem6 : Subsystem
  To Workspace : ToWorkspace  VariableName=EX20  SampleTime=-1
  wires:
  [PropertiesStream9] -> Subsystem2/1(Stream 9)
  [PropertiesStream13] -> Subsystem6/1(Stream 13)
  Subsystem1/1(B2) -> Bus Creator7/2
  Subsystem3/1(B4) -> Bus Creator7/4
  Subsystem5/1(B6) -> Bus Creator7/6
  Bus Creator7/1 -> To Workspace/1
  Subsystem/1(B1) -> Bus Creator7/1
  [PropertiesStream6] -> Subsystem/1(Stream 6)
  [PropertiesStream8] -> Subsystem1/1(Stream 8)
  Subsystem2/1(B3) -> Bus Creator7/3
  [PropertiesStream10] -> Subsystem3/1(Stream 10)
  Subsystem4/1(B5) -> Bus Creator7/5
  [PropertiesStream11] -> Subsystem4/1(Stream 11)
  [PropertiesStream5] -> Subsystem5/1(Stream 5)
  Subsystem6/1(B7) -> Bus Creator7/7

== system SP_Dynamic_17Okt_ExergyFlow/Valve ==
  Properties of Feed D : Inport
  Bus Creator : BusCreator  Inputs=5
  Bus Selector : BusSelector  OutputSignals=VRNG(1)
  Bus Selector1 : BusSelector  OutputSignals=XST(I;1),TST(1),HST(1)
  FCM(I,1) Component molar flow of Stream 1 lb-mol/h : Product  OutDataTypeStr=Inherit: Same as first input
  FTM(1) Total molar flow of Stream 1 lb-mol/h : Subsystem
  Position of Valve 1 % : Subsystem
  Properties of Stream 1 : Outport  VectorParamsAs1DForOutWhenUnconnected=off
  tag scope: PropertiesStream1=global
  wires:
  Position of Valve 1 %/1("YY(39) ") -> FTM(1) Total molar flow of Stream 1 lb-mol/h/1(VPOS(1))
  Properties of Feed D/1 -> Bus Selector1/1, Bus Selector/1
  Bus Selector/1 -> FTM(1) Total molar flow of Stream 1 lb-mol/h/2(VRNG(1))  "<VRNG(1)>"
  Bus Selector1/1 -> Bus Creator/1, FCM(I,1) Component molar flow of Stream 1 lb-mol/h/1  "<XST(I;1)>"
  FTM(1) Total molar flow of Stream 1 lb-mol/h/1(FTM(1)) -> Bus Creator/4, FCM(I,1) Component molar flow of Stream 1 lb-mol/h/2  "FTM(1)"
  Bus Selector1/2 -> Bus Creator/2  "<TST(1)>"
  Bus Selector1/3 -> Bus Creator/3  "<HST(1)>"
  FCM(I,1) Component molar flow of Stream 1 lb-mol/h/1 -> Bus Creator/5  "FCM(I;1)"
  Bus Creator/1 -> [PropertiesStream1], Properties of Stream 1/1

== system SP_Dynamic_17Okt_ExergyFlow/Valve 2 ==
  Properties of Feed E : Inport
  Bus Creator : BusCreator  Inputs=5
  Bus Selector : BusSelector  OutputSignals=VRNG(2)
  Bus Selector1 : BusSelector  OutputSignals=XST(I;2),TST(2),HST(2)
  FCM(I,2) Component molar flow of Stream 2 lb-mol/h : Product
  FTM(2) Total molar flow of Stream 2 lb-mol/h : Subsystem
  Position of Valve 2 % : Subsystem
  Properties of Stream 2 : Outport  VectorParamsAs1DForOutWhenUnconnected=off
  tag scope: PropertiesStream2=global
  wires:
  Properties of Feed E/1 -> Bus Selector1/1, Bus Selector/1
  Bus Selector/1 -> FTM(2) Total molar flow of Stream 2 lb-mol/h/2(VRNG(2))  "<VRNG(2)>"
  Bus Selector1/1 -> Bus Creator/1, FCM(I,2) Component molar flow of Stream 2 lb-mol/h/1  "<XST(I;2)>"
  FTM(2) Total molar flow of Stream 2 lb-mol/h/1(FTM(2)) -> Bus Creator/4, FCM(I,2) Component molar flow of Stream 2 lb-mol/h/2  "FTM(2)"
  Bus Selector1/2 -> Bus Creator/2  "<TST(2)>"
  Bus Selector1/3 -> Bus Creator/3  "<HST(2)>"
  FCM(I,2) Component molar flow of Stream 2 lb-mol/h/1 -> Bus Creator/5  "FCM(I;2)"
  Bus Creator/1 -> [PropertiesStream2], Properties of Stream 2/1
  Position of Valve 2 %/1("YY(40)  ") -> FTM(2) Total molar flow of Stream 2 lb-mol/h/1(VPOS(2))

== system SP_Dynamic_17Okt_ExergyFlow/Valve 3 ==
  Properties of Feed A : Inport
  Bus Creator : BusCreator  Inputs=5
  Bus Selector : BusSelector  OutputSignals=VRNG(3)
  Bus Selector1 : BusSelector  OutputSignals=XST(I;3),TST(3),HST(3)
  FCM(I,3) Component molar flow of Stream 3 lb-mol/h : Product
  FTM(3) Total molar flow of Stream 3 lb-mol/h : Subsystem
  Position of Valve 3 % : Subsystem
  Properties of Stream 3 : Outport  VectorParamsAs1DForOutWhenUnconnected=off
  tag scope: PropertiesStream3=global
  wires:
  Properties of Feed A/1 -> Bus Selector1/1, Bus Selector/1
  Bus Selector/1 -> FTM(3) Total molar flow of Stream 3 lb-mol/h/2(VRNG(3))  "<VRNG(3)>"
  Bus Selector1/1 -> Bus Creator/1, FCM(I,3) Component molar flow of Stream 3 lb-mol/h/1  "<XST(I;3)>"
  FTM(3) Total molar flow of Stream 3 lb-mol/h/1(FTM(3)) -> Bus Creator/4, FCM(I,3) Component molar flow of Stream 3 lb-mol/h/2  "FTM(3)"
  Bus Selector1/2 -> Bus Creator/2  "<TST(3)>"
  Bus Selector1/3 -> Bus Creator/3  "<HST(3)>"
  FCM(I,3) Component molar flow of Stream 3 lb-mol/h/1 -> Bus Creator/5  "FCM(I;3)"
  Bus Creator/1 -> [PropertiesStream3], Properties of Stream 3/1
  Position of Valve 3 %/1("YY(41) ") -> FTM(3) Total molar flow of Stream 3 lb-mol/h/1(VPOS(3))

== system SP_Dynamic_17Okt_ExergyFlow/Valve 4 ==
  Properties of Feed C : Inport
  Bus Creator : BusCreator  Inputs=5
  Bus Selector : BusSelector  OutputSignals=VRNG(4)
  Bus Selector1 : BusSelector  OutputSignals=XST(I;4),TST(4),HST(4)
  FCM(I,4) Component molar flow of Stream 4 lb-mol/h : Product
  FTM(4) Total molar flow of Stream 4 lb-mol/h : Subsystem
  Position of Valve 4 % : Subsystem
  Properties of Stream 4 : Outport  VectorParamsAs1DForOutWhenUnconnected=off
  tag scope: PropertiesStream4=global
  wires:
  Properties of Feed C/1 -> Bus Selector1/1, Bus Selector/1
  Bus Selector/1 -> FTM(4) Total molar flow of Stream 4 lb-mol/h/2(VRNG(4))  "<VRNG(4)>"
  Bus Selector1/1 -> Bus Creator/1, FCM(I,4) Component molar flow of Stream 4 lb-mol/h/1  "<XST(I;4)>"
  FTM(4) Total molar flow of Stream 4 lb-mol/h/1(FTM(4)) -> Bus Creator/4, FCM(I,4) Component molar flow of Stream 4 lb-mol/h/2  "FTM(4)"
  Bus Selector1/2 -> Bus Creator/2  "<TST(4)>"
  Bus Selector1/3 -> Bus Creator/3  "<HST(4)>"
  FCM(I,4) Component molar flow of Stream 4 lb-mol/h/1 -> Bus Creator/5  "FCM(I;4)"
  Bus Creator/1 -> [PropertiesStream4], Properties of Stream 4/1
  Position of Valve 4 %/1("YY(42) ") -> FTM(4) Total molar flow of Stream 4 lb-mol/h/1(VPOS(4))

== system SP_Dynamic_17Okt_ExergyFlow/Compressor/   ==
  PR : Inport
  CPFLMX : Inport  Port=2
  FLCOEF : Inport  Port=3
  " " : Constant
  "   " : Constant  Value=3
  Add : Sum
  Display : Display
  Display1 : Display
  Math Function : Math  Operator=pow  SaturateOnIntegerOverflow=on
  Product : Product
  Subtract : Sum  Inputs=+-
  FLMS : Outport  VectorParamsAs1DForOutWhenUnconnected=off
  wires:
  CPFLMX/1 -> Add/1
  Math Function/1 -> Subtract/2
  PR/1 -> Math Function/1
  " "/1 -> Subtract/1
  Add/1 -> Display1/1, FLMS/1
  FLCOEF/1 -> Display/1, Product/2
  "   "/1 -> Math Function/2
  Product/1 -> Add/2
  Subtract/1 -> Product/1

== system SP_Dynamic_17Okt_ExergyFlow/Compressor/CPDH Compressor work MBtu//h ==
  FLMS : Inport
  TKS : Inport  Port=2
  "XMWS(9) " : Inport  Port=3
  "Convert Btu/°R to MBtu/K " : Constant  Value=1.8e-6
  Divide : Product  Inputs=*/
  PTV-PTS : Sum  Inputs=+-
  Product : Product  Inputs=5
  Product1 : Product
  Universal gas constant Btu/lb-mol·°R : Constant  Value=1.9872
  CPDH : Outport  PortDimensions=1  VectorParamsAs1DForOutWhenUnconnected=off
  wires:
  "Convert Btu/°R to MBtu/K "/1 -> Product/3
  [PTS] -> Product1/2, PTV-PTS/2
  TKS/1 -> Product/2
  Universal gas constant Btu/lb-mol·°R/1 -> Product/4
  Product1/1 -> Divide/2
  Product/1 -> Divide/1
  PTV-PTS/1 -> Product/5
  FLMS/1 -> Product/1
  "XMWS(9) "/1 -> Product1/1
  [PTV] -> PTV-PTS/1
  Divide/1 -> CPDH/1

== system SP_Dynamic_17Okt_ExergyFlow/Compressor/Subsystem ==
  CPPRMX : Constant  Value=1.3
  Display : Display
  If : If  IfExpression=u1 < 1  ElseIfExpressions=u1>1.3
  If Action Subsystem : Subsystem  TreatAsAtomicUnit=on
  If Action Subsystem1 : Subsystem  TreatAsAtomicUnit=on
  If Action Subsystem2 : Subsystem  TreatAsAtomicUnit=on
  Merge : Merge  Inputs=3
  Minimum Pressure Ratio : Constant
  PR Pressure Ratio : Product  Inputs=*/
  PR : Outport  VectorParamsAs1DForOutWhenUnconnected=off
  wires:
  [PTS] -> PR Pressure Ratio/2
  PR Pressure Ratio/1 -> If Action Subsystem2/1(In1), If/1
  [PTV] -> PR Pressure Ratio/1
  If Action Subsystem1/1(Out1) -> Merge/2
  If Action Subsystem/1(Out1) -> Merge/1
  If/3 -> If Action Subsystem2/Action
  CPPRMX/1 -> If Action Subsystem1/1(In1)
  Minimum Pressure Ratio/1 -> If Action Subsystem/1(In1)
  If/2 -> If Action Subsystem1/Action
  If/1 -> If Action Subsystem/Action
  If Action Subsystem2/1(Out1) -> Merge/3
  Merge/1 -> Display/1, PR/1

== system SP_Dynamic_17Okt_ExergyFlow/Compressor/Subsystem1 ==
  CPFLMX : Inport
  " " : Constant  Value=1.197
  Divide : Product  Inputs=*/
  FLCOEF : Outport  VectorParamsAs1DForOutWhenUnconnected=off
  wires:
  " "/1 -> Divide/2
  Divide/1 -> FLCOEF/1
  CPFLMX/1 -> Divide/1

== system SP_Dynamic_17Okt_ExergyFlow/Condenser/FWS Flow of cooling water to Condenser lb-mol//h ==
  VPOS(11) : Inport
  VRNG(11) : Inport  Port=2
  " " : Product  Inputs=**/
  Constant2 : Constant  Value=100
  FWS : Outport  VectorParamsAs1DForOutWhenUnconnected=off
  wires:
  Constant2/1 -> " "/3
  " "/1 -> FWS/1
  VPOS(11)/1 -> " "/1
  VRNG(11)/1 -> " "/2

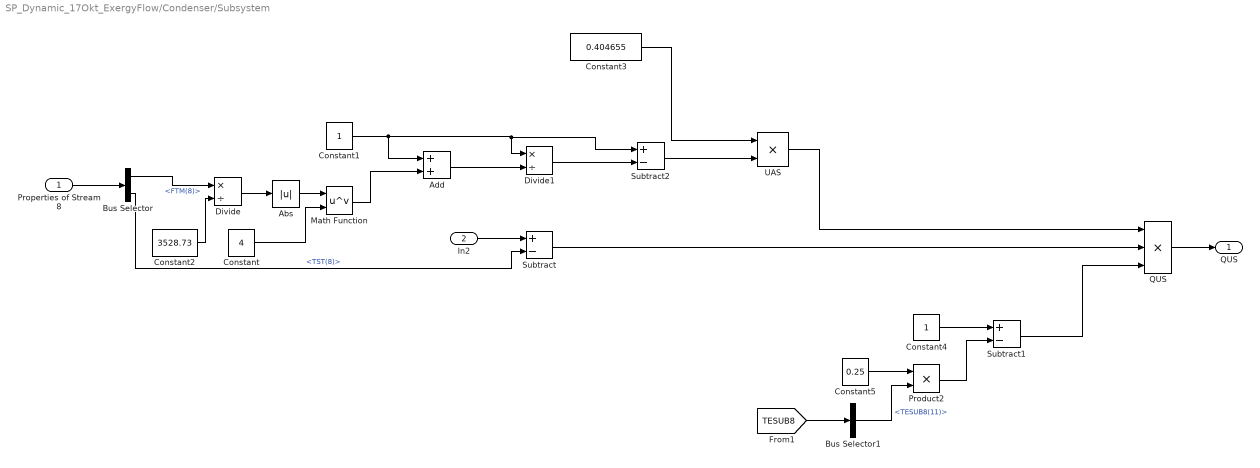
== system SP_Dynamic_17Okt_ExergyFlow/Condenser/Subsystem ==
  Properties of Stream 8 : Inport
  In2 : Inport  Port=2
  Abs : Abs
  Add : Sum
  Bus Selector : BusSelector  OutputSignals=FTM(8),TST(8)
  Bus Selector1 : BusSelector  OutputSignals=TESUB8(11)
  Constant : Constant  Value=4
  Constant1 : Constant
  Constant2 : Constant  Value=3528.73
  Constant3 : Constant  Value=0.404655
  Constant4 : Constant
  Constant5 : Constant  Value=0.25
  Divide : Product  Inputs=*/
  Divide1 : Product  Inputs=*/
  Math Function : Math  Operator=pow  SaturateOnIntegerOverflow=on
  Product2 : Product
  QUS : Product  Inputs=3
  Subtract : Sum  Inputs=+-
  Subtract1 : Sum  Inputs=+-
  Subtract2 : Sum  Inputs=+-
  UAS : Product
  "QUS " : Outport  VectorParamsAs1DForOutWhenUnconnected=off
  wires:
  Product2/1 -> Subtract1/2
  Constant4/1 -> Subtract1/1
  UAS/1 -> QUS/1
  Properties of Stream 8/1 -> Bus Selector/1
  Add/1 -> Divide1/2
  Constant2/1 -> Divide/2
  Math Function/1 -> Add/2
  Constant1/1 -> Subtract2/1, Divide1/1, Add/1
  Subtract1/1 -> QUS/3
  Constant/1 -> Math Function/2
  Bus Selector/2 -> Subtract/2  "<TST(8)>"
  Bus Selector/1 -> Divide/1  "<FTM(8)>"
  Divide1/1 -> Subtract2/2
  Divide/1 -> Abs/1
  Subtract/1 -> QUS/2
  Constant3/1 -> UAS/1
  Bus Selector1/1 -> Product2/2  "<TESUB8(11)>"
  Subtract2/1 -> UAS/2
  Constant5/1 -> Product2/1
  Abs/1 -> Math Function/1
  [TESUB8] -> Bus Selector1/1
  In2/1 -> Subtract/1
  QUS/1 -> "QUS "/1

== system SP_Dynamic_17Okt_ExergyFlow/Condenser/Subsystem1 ==
  FWS : Inport
  QUS : Inport  Port=2
  Constant1 : Constant  Value=1e6
  Constant2 : Constant  Value=1.8
  Constant6 : Constant  Value=500.53
  Divide : Product  Inputs=*/
  Divide1 : Product
  Divide2 : Product  Inputs=*/
  HWS : Constant  Value=11138
  Product : Product  Inputs=3
  Subtract : Sum  Inputs=+-
  TCWS : Subsystem
  TCWS-TWS : Sum  Inputs=+-
  YP(38) : Integrator  InitialConditionSource=external
  YY(38) : Constant  Value=77.29698353
  "YY(38) " : Outport  VectorParamsAs1DForOutWhenUnconnected=off
  tag scope: TWS=global
  wires:
  Divide2/1 -> YP(38)/1
  YY(38)/1 -> YP(38)/2
  TCWS/1(TCWS) -> TCWS-TWS/1
  YP(38)/1 -> [TWS], "YY(38) "/1, TCWS-TWS/2
  FWS/1 -> Product/1
  Constant6/1 -> Product/2
  TCWS-TWS/1 -> Product/3
  QUS/1 -> Divide1/1
  Constant1/1 -> Divide1/2
  Divide1/1 -> Divide/1
  Constant2/1 -> Divide/2
  Product/1 -> Subtract/1
  Divide/1 -> Subtract/2
  Subtract/1 -> Divide2/1
  HWS/1 -> Divide2/2

== system SP_Dynamic_17Okt_ExergyFlow/D Feed Stream 1/HST(1) Molar Enthalpy of Stream 1 MBtu//lb-mol ==
  TST(1) : Inport
  XST(I,1) : Inport  Port=2
  "Enthalpy of Stream " : mylib/Enthalpy of Stream   SystemSampleTime=-1  Latency=0  AutoFrameSizeCalculation=off
  ITY : Constant
  HST(1) : Outport  VectorParamsAs1DForOutWhenUnconnected=off
  wires:
  ITY/1 -> "Enthalpy of Stream "/1
  TST(1)/1 -> "Enthalpy of Stream "/2
  XST(I,1)/1 -> "Enthalpy of Stream "/3
  "Enthalpy of Stream "/1 -> HST(1)/1

== system SP_Dynamic_17Okt_ExergyFlow/D Feed Stream 1/TST(1) Temperature of Stream 1 °C ==
  Add : Sum
  Bus Selector : BusSelector  OutputSignals=TESUB8(3)
  Bus Selector1 : BusSelector  OutputSignals=IDV(3)
  Constant : Constant  Value=5
  Product : Product
  TST(1) : Outport  PortDimensions=1  VectorParamsAs1DForOutWhenUnconnected=off
  wires:
  Constant/1 -> Product/2
  Bus Selector1/1 -> Product/1  "<IDV(3)>"
  [IDV] -> Bus Selector1/1
  [TESUB8] -> Bus Selector/1
  Add/1 -> TST(1)/1  "TST(1)"
  Product/1 -> Add/2
  Bus Selector/1 -> Add/1  "<TESUB8(3)>"

== system SP_Dynamic_17Okt_ExergyFlow/D Feed Stream 2/HST(2) Molar Enthalpy of Stream 2 MBtu//lb-mol ==
  TST(2) : Inport
  XST(I,2) : Inport  Port=2
  "Enthalpy of Stream " : mylib/Enthalpy of Stream   SystemSampleTime=-1  Latency=0  AutoFrameSizeCalculation=off
  ITY : Constant
  HST(2) : Outport  VectorParamsAs1DForOutWhenUnconnected=off
  wires:
  ITY/1 -> "Enthalpy of Stream "/1
  TST(2)/1 -> "Enthalpy of Stream "/2
  XST(I,2)/1 -> "Enthalpy of Stream "/3
  "Enthalpy of Stream "/1 -> HST(2)/1

== system SP_Dynamic_17Okt_ExergyFlow/D Feed Stream 3/HST(3) Molar Enthalpy of Stream 3 MBtu//lb-mol ==
  TST(3) : Inport
  XST(I,3) : Inport  Port=2
  "Enthalpy of Stream " : mylib/Enthalpy of Stream   SystemSampleTime=-1  Latency=0  AutoFrameSizeCalculation=off
  ITY : Constant
  HST(3) : Outport  VectorParamsAs1DForOutWhenUnconnected=off
  wires:
  ITY/1 -> "Enthalpy of Stream "/1
  TST(3)/1 -> "Enthalpy of Stream "/2
  XST(I,3)/1 -> "Enthalpy of Stream "/3
  "Enthalpy of Stream "/1 -> HST(3)/1
